simulink model "HMI_C_S_28379D_071224_FW"  (R2024b)
settings: Solver=ode4  StartTime=0.0  StopTime=Inf  FixedStep=Ts  RelTol=1e-3  EnableMultiTasking=on
InitFcn:
  | Ts=1e-4
model workspace (MAT data in the model file):
  encoderResolution = 2000
  hallOffset = '0.5'
  indexOffset = 850
  polePairs = '4'
libraries: simulink x4, c2837xDlib x2, c280xlib x2
settings Model: ExtModeTrigDuration=8  Creator=matti  LastModifiedBy=Administrator
settings SolverCC: AlgebraicLoopSolver=TrustRegion
settings DataIOCC: LimitDataPoints=on  SaveFormat=Array  SignalLoggingSaveFormat=ModelDataLogs  SaveOutput=off  SaveTime=off  ReturnWorkspaceOutputs=off
settings OptimizationCC: DefaultUnderspecifiedDataType=single  OptimizeBlockIOStorage=off  BufferReuse=off  GlobalBufferReuse=off  ExpressionFolding=off  ExpressionDepthLimit=2147483647  LocalBlockOutputs=off  InitFltsAndDblsToZero=on  NoFixptDivByZeroProtection=on  EfficientFloat2IntCast=on  EfficientMapNaN2IntZero=off  LifeSpan=Inf  MaxStackSize=1024  OptimizeDataStoreBuffers=off  BusAssignmentInplaceUpdate=off  EfficientTunableParamExpr=on
settings DebuggingCC: ReadBeforeWriteMsg=DisableAll  WriteAfterWriteMsg=DisableAll  WriteAfterReadMsg=DisableAll  CheckSSInitialOutputMsg=off  UnderspecifiedInitializationDetection=Classic  MergeDetectMultiDrivingBlocksExec=none  SignalResolutionControl=TryResolveAllWithWarning  SolverPrmCheckMsg=warning  InheritedTsInSrcMsg=none  MultiTaskDSMMsg=none  MultiTaskCondExecSysMsg=none  TasksWithSamePriorityMsg=none  SigSpecEnsureSampleTimeMsg=none  IntegerOverflowMsg=none  ParameterPrecisionLossMsg=none  FcnCallInpInsideContextMsg=warning  UnconnectedInputMsg=warning  UnconnectedOutputMsg=warning  UnconnectedLineMsg=warning  StateNameClashWarn=warning  SFUnexpectedBacktrackingDiag=warning  SFNoUnconditionalDefaultTransitionDiag=warning  SFExecutionAtInitializationDiag=none  IntegerSaturationMsg=none  ArithmeticOperatorsInVariantConditions=warning
settings HardwareCC: ProdBitPerChar=16  ProdBitPerInt=16  ProdBitPerPointer=32  ProdBitPerSizeT=32  ProdBitPerPtrDiffT=32  ProdLargestAtomicInteger=Integer  ProdLargestAtomicFloat=None  ProdWordSize=16  ProdLongLongMode=on  ProdHWDeviceType=Texas Instruments->C2000  TargetBitPerChar=16  TargetBitPerInt=16  TargetBitPerPointer=16  TargetLargestAtomicInteger=Integer  TargetIntDivRoundTo=Zero  TargetEndianess=LittleEndian  TargetWordSize=16  TargetHWDeviceType=TI C2000  HardwareBoardFeatureSet=SoCBlockset
settings ModelReferenceCC: EnableRefExpFcnMdlSchedulingChecks=on  PropagateSignalLabelsOutOfModel=off
settings SFSimCC: SimUseLocalCustomCode=off  MATLABDynamicMemAlloc=off  CustomCodeUndefinedFunction=UseInterfaceOnly
settings RTWCC: Description=Embedded Coder  SystemTargetFile=ert.tlc  HardwareBoard=TI Delfino F28379D LaunchPad  TemplateMakefile=ert_default_tmf  GenerateReport=on  RTWUseLocalCustomCode=off  CustomHeaderCode=#include<stdlib.h>  Toolchain=Texas Instruments Code Composer Studio (C2000)  IncludeHyperlinkInReport=on  LaunchReport=on  CodeProfilingSaveOptions=MetricsOnly  GenerateTraceInfo=on  GenerateTraceReport=on  GenerateTraceReportSl=on  GenerateTraceReportSf=on  GenerateTraceReportEml=on  GPUComputeCapability=3.5
settings CodeAppCC: IgnoreCustomStorageClasses=off  CustomSymbolStrType=$N$R$M  StateflowObjectComments=on  InternalIdentifier=Classic
settings ERTTargetCC: CodeReplacementLibrary=TI C28x  MultiwordLength=2048  SupportContinuousTime=on  ExtModeTransport=4  ExtModeStaticAlloc=on  ExtModeAutomaticAllocSize=off  ExtModeStaticAllocSize=10000  ExtModeMexFile=ext_xcp  ExtModeIntrfLevel=Level2 - Open  InlinedParameterPlacement=Hierarchical  ConvertIfToSwitch=off  SuppressUnreachableDefaultCases=off  MemSecPackage=tic2000demospkg  MemSecFuncExecute=code_ramfuncs  DynamicArrayContainerType=coder::array
settings ConfigComp: CovMetricSettings=dw  CovSaveCumulativeToWorkspaceVar=on  CovSaveSingleToWorkspaceVar=on  CovExternalEMLEnable=off  CovSFcnEnable=off
settings SimscapeCC: SimscapeNormalizeSystem=off

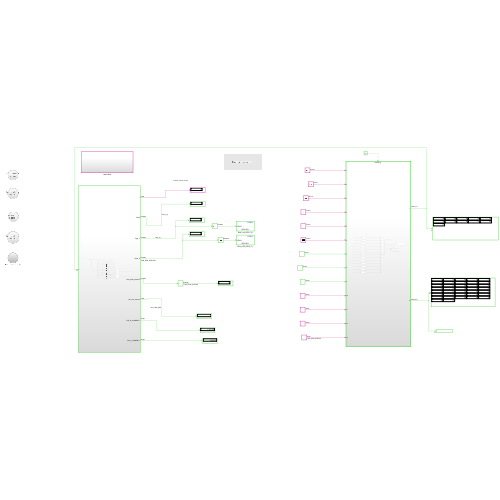
[thumbnail: Simulink's stored preview of the top-level diagram]
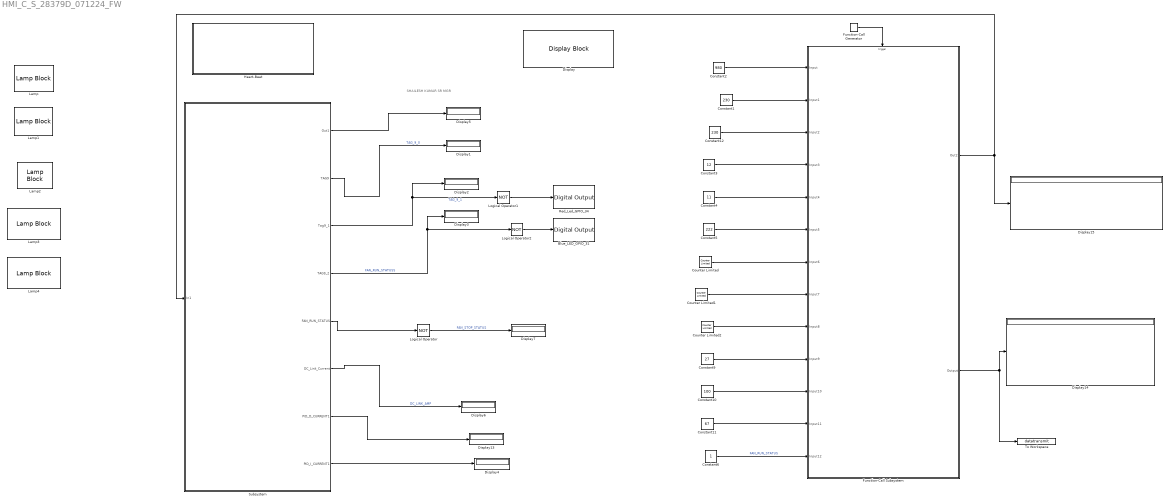
== system HMI_C_S_28379D_071224_FW ==
  note: SHAILESH KUMAR SR MGR
  Blue_LED_GPIO_31 : c2837xDlib/Digital Output  GPIO_Number=GPIO24~GPIO31  GPIO_Bit0=off  GPIO_BIT0_Toggle=off  GPIO_Bit1=off  GPIO_BIT1_Toggle=off  GPIO_Bit2=off  GPIO_BIT2_Toggle=off  GPIO_Bit3=off  GPIO_BIT3_Toggle=off  GPIO_Bit4=off  GPIO_BIT4_Toggle=off  GPIO_Bit5=off  GPIO_BIT5_Toggle=off  GPIO_Bit6=off  GPIO_BIT6_Toggle=off  GPIO_Bit7=on  GPIO_BIT7_Toggle=off
  Constant1 : Constant  Value=230  OutDataTypeStr=uint16
  Constant10 : Constant  Value=100  OutDataTypeStr=uint16
  Constant11 : Constant  Value=67  OutDataTypeStr=uint16
  Constant12 : Constant  Value=230  OutDataTypeStr=uint16
  Constant2 : Constant  Value=980  OutDataTypeStr=uint16
  Constant3 : Constant  Value=12  OutDataTypeStr=uint16
  Constant4 : Constant  Value=11  OutDataTypeStr=uint16
  Constant5 : Constant  Value=222  OutDataTypeStr=uint16
  Constant6 : Constant  OutDataTypeStr=uint8
  Constant9 : Constant  Value=27  OutDataTypeStr=uint16
  Counter Limited : simulink/Sources/Counter Limited  uplimit=999  tsamp=-1
  Counter Limited1 : simulink/Sources/Counter Limited  uplimit=999  tsamp=-1
  Counter Limited2 : simulink/Sources/Counter Limited  uplimit=999  tsamp=-1
  Display : DisplayBlock  Transparency=1
  Display{1..7,13..15} (10 alike) : Display
  Function-Call Generator : simulink/Ports & Subsystems/Function-Call Generator  sample_time=0.1  numberOfIterations=1  DisallowWideOutput=off
  Function-Call Subsystem : Subsystem  TreatAsAtomicUnit=on
  Heart-Beat : Subsystem
  Lamp : LampBlock
  Lamp1 : LampBlock
  Lamp2 : LampBlock
  Lamp3 : LampBlock  LabelPosition=Bottom
  Lamp4 : LampBlock  LabelPosition=Bottom
  Logical Operator : Logic  Operator=NOT  AllPortsSameDT=off  OutDataTypeStr=boolean
  Logical Operator1 : Logic  Operator=NOT  AllPortsSameDT=off  OutDataTypeStr=boolean
  Logical Operator2 : Logic  Operator=NOT  AllPortsSameDT=off  OutDataTypeStr=boolean
  Red_Led_GPIO_34 : c2837xDlib/Digital Output  GPIO_Number=GPIO32~GPIO39  GPIO_Bit0=off  GPIO_BIT0_Toggle=off  GPIO_Bit1=off  GPIO_BIT1_Toggle=off  GPIO_Bit2=on  GPIO_BIT2_Toggle=off  GPIO_Bit3=off  GPIO_BIT3_Toggle=off  GPIO_Bit4=off  GPIO_BIT4_Toggle=off  GPIO_Bit5=off  GPIO_BIT5_Toggle=off  GPIO_Bit6=off  GPIO_BIT6_Toggle=off  GPIO_Bit7=off  GPIO_BIT7_Toggle=off
  Subsystem : Subsystem
  To Workspace : ToWorkspace  VariableName=datatransmit  SampleTime=-1
      settings: Save2DSignal=2-D array (concatenate along first dimension)
  wires:
  Subsystem/1(Out1) -> Display5/1
  Subsystem/3(Tag9_1) -> Display2/1, Logical Operator1/1  "TAG_9_1"
  Subsystem/6(DC_Link_Current) -> Display6/1  "DC_LINK_AMP"
  Subsystem/2(TAG9) -> Display1/1  "TAG_9_0"
  Logical Operator/1 -> Display7/1  "FAN_STOP_STATUS"
  Function-Call Generator/1 -> Function-Call Subsystem/Trigger
  Function-Call Subsystem/1(Out2) -> Subsystem/1(In1), Display15/1
  Constant2/1 -> Function-Call Subsystem/1(Input)
  Constant1/1 -> Function-Call Subsystem/2(Input1)
  Constant12/1 -> Function-Call Subsystem/3(Input2)
  Constant3/1 -> Function-Call Subsystem/4(Input3)
  Constant4/1 -> Function-Call Subsystem/5(Input4)
  Constant5/1 -> Function-Call Subsystem/6(Input5)
  Counter Limited/1 -> Function-Call Subsystem/7(Input6)
  Counter Limited1/1 -> Function-Call Subsystem/8(Input7)
  Counter Limited2/1 -> Function-Call Subsystem/9(Input8)
  Constant9/1 -> Function-Call Subsystem/10(Input9)
  Constant10/1 -> Function-Call Subsystem/11(Input10)
  Constant11/1 -> Function-Call Subsystem/12(Input11)
  Constant6/1 -> Function-Call Subsystem/13(Input12)  "FAN_RUN_STATUS"
  Function-Call Subsystem/2(Output) -> To Workspace/1, Display14/1
  Logical Operator1/1 -> Red_Led_GPIO_34/1
  Logical Operator2/1 -> Blue_LED_GPIO_31/1
  Subsystem/4(TAG9_2) -> Display3/1, Logical Operator2/1  "FAN_RUN_STATUSS"
  Subsystem/5(FAN_RUN_STATUS) -> Logical Operator/1
  Subsystem/7(PID_D_CURRENT1) -> Display13/1
  Subsystem/8(PID_I_CURRENT1) -> Display4/1

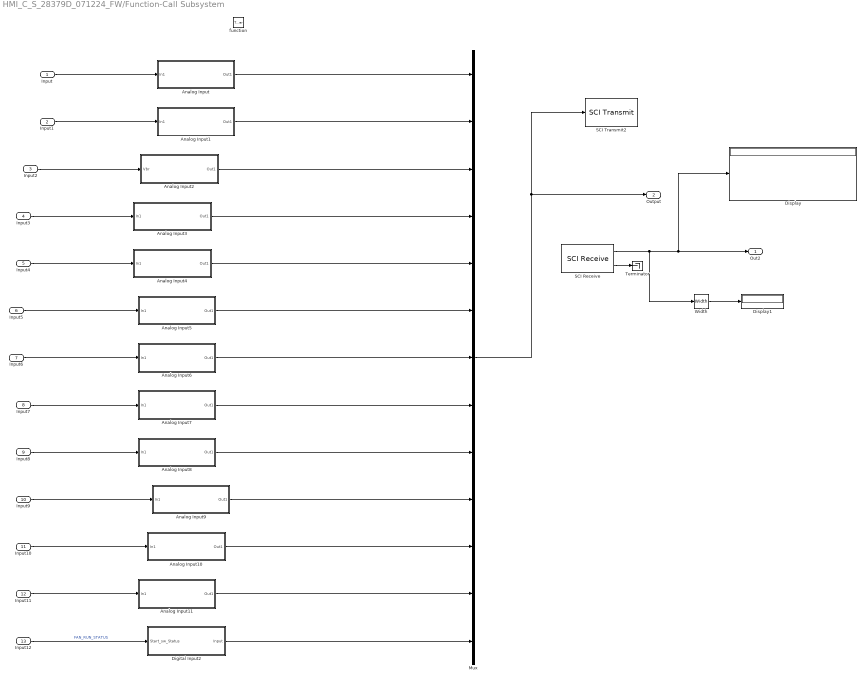
== system HMI_C_S_28379D_071224_FW/Function-Call Subsystem ==
  Input : Inport
  Input1 : Inport  Port=2
  Input2 : Inport  Port=3
  Input3 : Inport  Port=4
  Input4 : Inport  Port=5
  Input5 : Inport  Port=6
  Input6 : Inport  Port=7
  Input7 : Inport  Port=8
  Input8 : Inport  Port=9
  Input9 : Inport  Port=10
  Input10 : Inport  Port=11
  Input11 : Inport  Port=12
  Input12 : Inport  Port=13
  function : TriggerPort  TriggerType=function-call  VariantControl=(inherit)
  Analog Input : Subsystem
  Analog Input1 : Subsystem
  Analog Input10 : Subsystem
  Analog Input11 : Subsystem
  Analog Input2 : Subsystem
  Analog Input3 : Subsystem
  Analog Input4 : Subsystem
  Analog Input5 : Subsystem
  Analog Input6 : Subsystem
  Analog Input7 : Subsystem
  Analog Input8 : Subsystem
  Analog Input9 : Subsystem
  Digital Input2 : Subsystem
  Display : Display
  Display1 : Display
  Mux : Mux  Inputs=13
  SCI Receive : c280xlib/SCI Receive  Priority=2  sciModule=B  dataHead='S'  headerCheckMaxCount=16  dataTail='E'  dataType=uint8  dataLenOptions=Length via dialog  dataDim=11  maxDataLength=1  initValue=0  errOption=Output the last received value  errValue=0  sampleTime=-1  blockingMode=off  timeOut=inf  outputStatus=on
      settings: LibrarySourceBlock=c2837xDlib/SCI Receive
  SCI Transmit2 : c280xlib/SCI Transmit  sciModule=B  dataHead='S'  dataTail='E'  frameSize=[1 37]  blockingMode=on  outputStatus=off
      settings: LibrarySourceBlock=c2837xDlib/SCI Transmit
  Terminator : Terminator
  Width : Width  DataType=uint8
  Out2 : Outport
  Output : Outport  Port=2
  wires:
  SCI Receive/1 -> Width/1, Display/1, Out2/1
  SCI Receive/2 -> Terminator/1
  Analog Input1/1(Out1) -> Mux/2
  Analog Input2/1(Out1) -> Mux/3
  Analog Input9/1(Out1) -> Mux/10
  Analog Input7/1(Out1) -> Mux/8
  Analog Input4/1(Out1) -> Mux/5
  Analog Input5/1(Out1) -> Mux/6
  Digital Input2/1(Input) -> Mux/13
  Analog Input8/1(Out1) -> Mux/9
  Analog Input10/1(Out1) -> Mux/11
  Analog Input11/1(Out1) -> Mux/12
  Analog Input/1(Out1) -> Mux/1
  Input1/1 -> Analog Input1/1(In1)
  Input2/1 -> Analog Input2/1(Vbr)
  Input/1 -> Analog Input/1(In1)
  Input9/1 -> Analog Input9/1(In1)
  Input12/1 -> Digital Input2/1(Start_sw_Status)  "FAN_RUN_STATUS"
  Analog Input3/1(Out1) -> Mux/4
  Input11/1 -> Analog Input11/1(In1)
  Analog Input6/1(Out1) -> Mux/7
  Input10/1 -> Analog Input10/1(In1)
  Mux/1 -> SCI Transmit2/1, Output/1
  Input3/1 -> Analog Input3/1(In1)
  Input4/1 -> Analog Input4/1(In1)
  Input5/1 -> Analog Input5/1(In1)
  Input6/1 -> Analog Input6/1(In1)
  Input7/1 -> Analog Input7/1(In1)
  Input8/1 -> Analog Input8/1(In1)
  Width/1 -> Display1/1

== system HMI_C_S_28379D_071224_FW/Heart-Beat ==

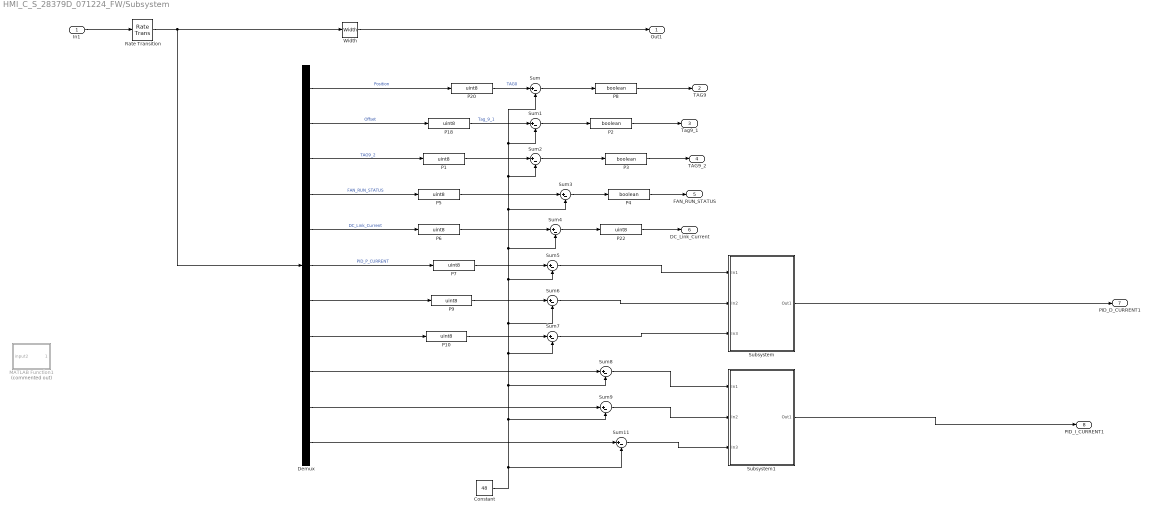
== system HMI_C_S_28379D_071224_FW/Subsystem ==
  In1 : Inport
  Constant : Constant  Value=48  OutDataTypeStr=uint8
  Demux : Demux  Outputs=11
  MATLAB Function1 : MATLAB Function  Commented=on  TreatAsAtomicUnit=on
  P{1,5..7,9..10,18,20,22} (9 alike) : DataTypeConversion  OutDataTypeStr=uint8  SaturateOnIntegerOverflow=off  RndMeth=Floor
  P{2..4,8} (4 alike) : DataTypeConversion  OutDataTypeStr=boolean  SaturateOnIntegerOverflow=off  RndMeth=Floor
  Rate Transition : RateTransition
  Subsystem : Subsystem
  Subsystem1 : Subsystem
  Sum{,1..9,11} (11 alike) : Sum  Inputs=|+-
  Width : Width  DataType=uint8
  Out1 : Outport
  TAG9 : Outport  Port=2
  Tag9_1 : Outport  Port=3
  TAG9_2 : Outport  Port=4
  FAN_RUN_STATUS : Outport  Port=5
  DC_Link_Current : Outport  Port=6
  PID_D_CURRENT1 : Outport  Port=7
  PID_I_CURRENT1 : Outport  Port=8
  wires:
  Demux/1 -> P20/1  "Position"
  P1/1 -> Sum2/1
  P3/1 -> TAG9_2/1
  Sum1/1 -> P2/1
  P10/1 -> Sum7/1
  P2/1 -> Tag9_1/1
  Sum/1 -> P8/1
  P18/1 -> Sum1/1  "Tag_9_1"
  P6/1 -> Sum4/1
  P9/1 -> Sum6/1
  P7/1 -> Sum5/1
  Demux/5 -> P6/1  "DC_Link_Current"
  Demux/6 -> P7/1  "PID_P_CURRENT"
  Demux/8 -> P10/1
  P4/1 -> FAN_RUN_STATUS/1
  Demux/4 -> P5/1  "FAN_RUN_STATUS"
  P5/1 -> Sum3/1
  Sum3/1 -> P4/1
  Demux/3 -> P1/1  "TAG9_2"
  Sum4/1 -> P22/1
  Demux/2 -> P18/1  "Offset"
  Sum2/1 -> P3/1
  In1/1 -> Rate Transition/1
  Width/1 -> Out1/1
  P20/1 -> Sum/1  "TAG0"
  Rate Transition/1 -> Demux/1, Width/1
  Demux/7 -> P9/1
  P8/1 -> TAG9/1
  P22/1 -> DC_Link_Current/1
  Constant/1 -> Sum11/2, Sum9/2, Sum8/2, Sum7/2, Sum6/2, Sum5/2, Sum4/2, Sum3/2, Sum2/2, Sum1/2, Sum/2
  Sum5/1 -> Subsystem/1(In1)
  Sum6/1 -> Subsystem/2(In2)
  Sum7/1 -> Subsystem/3(In3)
  Subsystem/1(Out1) -> PID_D_CURRENT1/1
  Demux/9 -> Sum8/1
  Demux/10 -> Sum9/1
  Demux/11 -> Sum11/1
  Sum11/1 -> Subsystem1/3(In3)
  Sum9/1 -> Subsystem1/2(In2)
  Sum8/1 -> Subsystem1/1(In1)
  Subsystem1/1(Out1) -> PID_I_CURRENT1/1

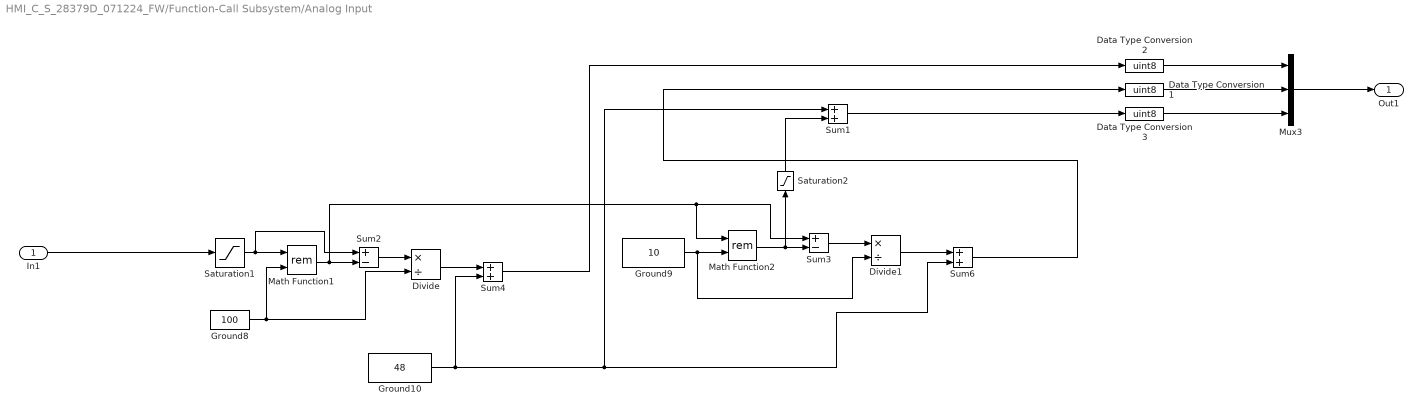
== system HMI_C_S_28379D_071224_FW/Function-Call Subsystem/Analog Input ==
  In1 : Inport
  Data Type Conversion1 : DataTypeConversion  OutDataTypeStr=uint8  SaturateOnIntegerOverflow=off  RndMeth=Floor
  Data Type Conversion2 : DataTypeConversion  OutDataTypeStr=uint8  SaturateOnIntegerOverflow=off  RndMeth=Floor
  Data Type Conversion3 : DataTypeConversion  OutDataTypeStr=uint8  SaturateOnIntegerOverflow=off  RndMeth=Floor
  Divide : Product  Inputs=*/  OutDataTypeStr=int16
  Divide1 : Product  Inputs=*/  OutDataTypeStr=int16
  Ground10 : Constant  Value=48  OutDataTypeStr=int16
  Ground8 : Constant  Value=100  OutDataTypeStr=int16
  Ground9 : Constant  Value=10  OutDataTypeStr=int16
  Math Function1 : Math  Operator=rem  SignedPower=on
  Math Function2 : Math  Operator=rem  SignedPower=on
  Mux3 : Mux  Inputs=3
  Saturation1 : Saturate  UpperLimit=999  LowerLimit=0  OutDataTypeStr=int16
  Saturation2 : Saturate  UpperLimit=9  LowerLimit=0
  Sum1 : Sum  OutDataTypeStr=uint8
  Sum2 : Sum  Inputs=+-  OutDataTypeStr=double
  Sum3 : Sum  Inputs=+-
  Sum4 : Sum  OutDataTypeStr=uint8
  Sum6 : Sum  OutDataTypeStr=uint8
  Out1 : Outport
  wires:
  Saturation1/1 -> Sum2/1, Math Function1/1
  Ground8/1 -> Divide/2, Math Function1/2
  Sum4/1 -> Data Type Conversion2/1
  Sum1/1 -> Data Type Conversion3/1
  Divide/1 -> Sum4/1
  Divide1/1 -> Sum6/1
  Sum2/1 -> Divide/1
  In1/1 -> Saturation1/1
  Data Type Conversion2/1 -> Mux3/1
  Mux3/1 -> Out1/1
  Data Type Conversion3/1 -> Mux3/3
  Data Type Conversion1/1 -> Mux3/2
  Math Function1/1 -> Sum2/2, Math Function2/1, Sum3/1
  Sum3/1 -> Divide1/1
  Sum6/1 -> Data Type Conversion1/1
  Ground10/1 -> Sum4/2, Sum6/2, Sum1/1
  Ground9/1 -> Divide1/2, Math Function2/2
  Math Function2/1 -> Sum3/2, Saturation2/1
  Saturation2/1 -> Sum1/2

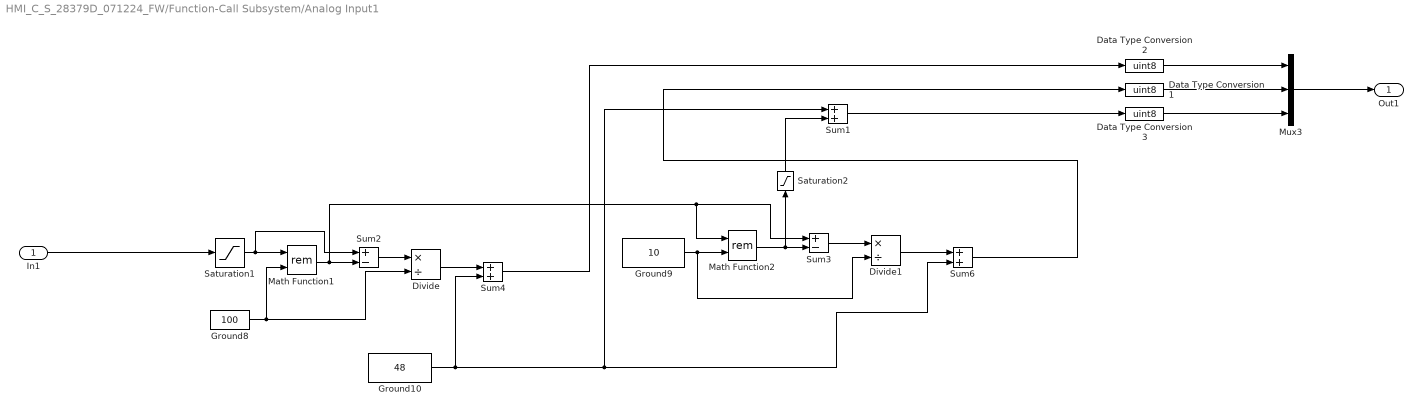
== system HMI_C_S_28379D_071224_FW/Function-Call Subsystem/Analog Input1 ==
  In1 : Inport
  Data Type Conversion1 : DataTypeConversion  OutDataTypeStr=uint8  SaturateOnIntegerOverflow=off  RndMeth=Floor
  Data Type Conversion2 : DataTypeConversion  OutDataTypeStr=uint8  SaturateOnIntegerOverflow=off  RndMeth=Floor
  Data Type Conversion3 : DataTypeConversion  OutDataTypeStr=uint8  SaturateOnIntegerOverflow=off  RndMeth=Floor
  Divide : Product  Inputs=*/  OutDataTypeStr=int16
  Divide1 : Product  Inputs=*/  OutDataTypeStr=int16
  Ground10 : Constant  Value=48  OutDataTypeStr=int16
  Ground8 : Constant  Value=100  OutDataTypeStr=int16
  Ground9 : Constant  Value=10  OutDataTypeStr=int16
  Math Function1 : Math  Operator=rem  SignedPower=on
  Math Function2 : Math  Operator=rem  SignedPower=on
  Mux3 : Mux  Inputs=3
  Saturation1 : Saturate  UpperLimit=999  LowerLimit=0  OutDataTypeStr=int16
  Saturation2 : Saturate  UpperLimit=9  LowerLimit=0
  Sum1 : Sum  OutDataTypeStr=uint8
  Sum2 : Sum  Inputs=+-  OutDataTypeStr=double
  Sum3 : Sum  Inputs=+-
  Sum4 : Sum  OutDataTypeStr=uint8
  Sum6 : Sum  OutDataTypeStr=uint8
  Out1 : Outport
  wires:
  Saturation1/1 -> Sum2/1, Math Function1/1
  Ground8/1 -> Divide/2, Math Function1/2
  Sum4/1 -> Data Type Conversion2/1
  Sum1/1 -> Data Type Conversion3/1
  Divide/1 -> Sum4/1
  Divide1/1 -> Sum6/1
  Sum2/1 -> Divide/1
  In1/1 -> Saturation1/1
  Data Type Conversion2/1 -> Mux3/1
  Mux3/1 -> Out1/1
  Data Type Conversion3/1 -> Mux3/3
  Data Type Conversion1/1 -> Mux3/2
  Math Function1/1 -> Sum2/2, Math Function2/1, Sum3/1
  Sum3/1 -> Divide1/1
  Sum6/1 -> Data Type Conversion1/1
  Ground10/1 -> Sum4/2, Sum6/2, Sum1/1
  Ground9/1 -> Divide1/2, Math Function2/2
  Math Function2/1 -> Sum3/2, Saturation2/1
  Saturation2/1 -> Sum1/2

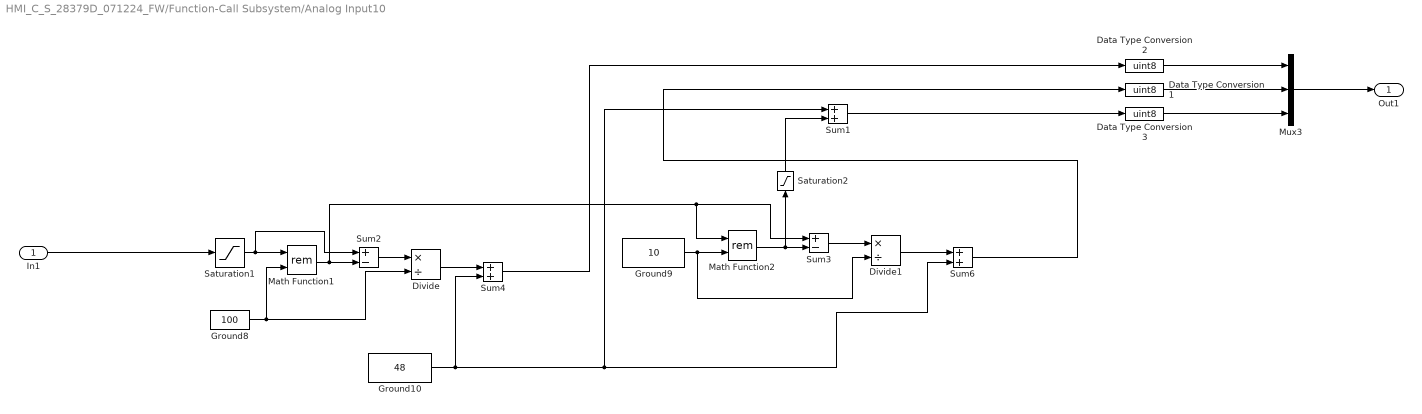
== system HMI_C_S_28379D_071224_FW/Function-Call Subsystem/Analog Input10 ==
  In1 : Inport
  Data Type Conversion1 : DataTypeConversion  OutDataTypeStr=uint8  SaturateOnIntegerOverflow=off  RndMeth=Floor
  Data Type Conversion2 : DataTypeConversion  OutDataTypeStr=uint8  SaturateOnIntegerOverflow=off  RndMeth=Floor
  Data Type Conversion3 : DataTypeConversion  OutDataTypeStr=uint8  SaturateOnIntegerOverflow=off  RndMeth=Floor
  Divide : Product  Inputs=*/  OutDataTypeStr=int16
  Divide1 : Product  Inputs=*/  OutDataTypeStr=int16
  Ground10 : Constant  Value=48  OutDataTypeStr=int16
  Ground8 : Constant  Value=100  OutDataTypeStr=int16
  Ground9 : Constant  Value=10  OutDataTypeStr=int16
  Math Function1 : Math  Operator=rem  SignedPower=on
  Math Function2 : Math  Operator=rem  SignedPower=on
  Mux3 : Mux  Inputs=3
  Saturation1 : Saturate  UpperLimit=999  LowerLimit=0  OutDataTypeStr=int16
  Saturation2 : Saturate  UpperLimit=9  LowerLimit=0
  Sum1 : Sum  OutDataTypeStr=uint8
  Sum2 : Sum  Inputs=+-  OutDataTypeStr=double
  Sum3 : Sum  Inputs=+-
  Sum4 : Sum  OutDataTypeStr=uint8
  Sum6 : Sum  OutDataTypeStr=uint8
  Out1 : Outport
  wires:
  Saturation1/1 -> Sum2/1, Math Function1/1
  Ground8/1 -> Divide/2, Math Function1/2
  Sum4/1 -> Data Type Conversion2/1
  Sum1/1 -> Data Type Conversion3/1
  Divide/1 -> Sum4/1
  Divide1/1 -> Sum6/1
  Sum2/1 -> Divide/1
  In1/1 -> Saturation1/1
  Data Type Conversion2/1 -> Mux3/1
  Mux3/1 -> Out1/1
  Data Type Conversion3/1 -> Mux3/3
  Data Type Conversion1/1 -> Mux3/2
  Math Function1/1 -> Sum2/2, Math Function2/1, Sum3/1
  Sum3/1 -> Divide1/1
  Sum6/1 -> Data Type Conversion1/1
  Ground10/1 -> Sum4/2, Sum6/2, Sum1/1
  Ground9/1 -> Divide1/2, Math Function2/2
  Math Function2/1 -> Sum3/2, Saturation2/1
  Saturation2/1 -> Sum1/2

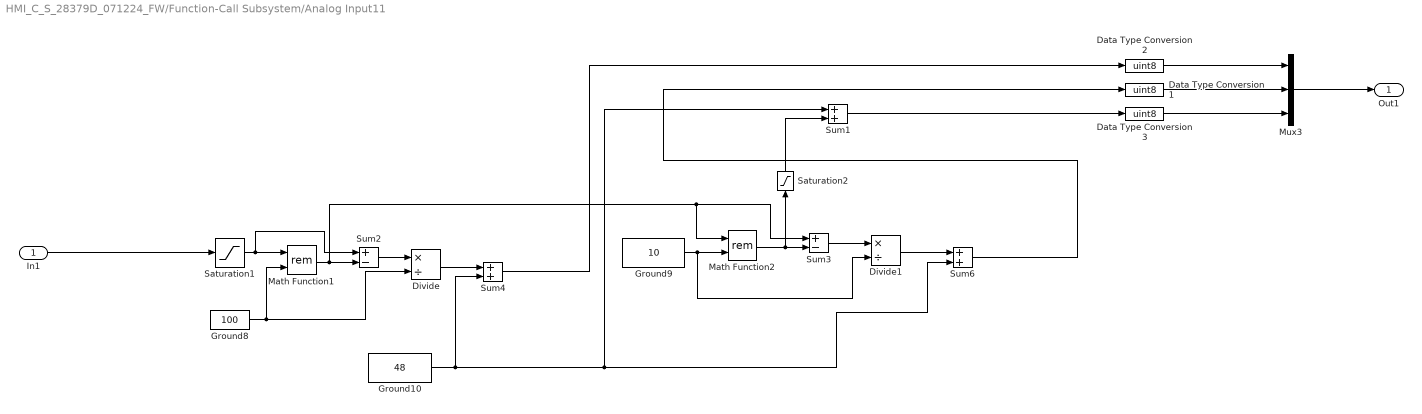
== system HMI_C_S_28379D_071224_FW/Function-Call Subsystem/Analog Input11 ==
  In1 : Inport
  Data Type Conversion1 : DataTypeConversion  OutDataTypeStr=uint8  SaturateOnIntegerOverflow=off  RndMeth=Floor
  Data Type Conversion2 : DataTypeConversion  OutDataTypeStr=uint8  SaturateOnIntegerOverflow=off  RndMeth=Floor
  Data Type Conversion3 : DataTypeConversion  OutDataTypeStr=uint8  SaturateOnIntegerOverflow=off  RndMeth=Floor
  Divide : Product  Inputs=*/  OutDataTypeStr=int16
  Divide1 : Product  Inputs=*/  OutDataTypeStr=int16
  Ground10 : Constant  Value=48  OutDataTypeStr=int16
  Ground8 : Constant  Value=100  OutDataTypeStr=int16
  Ground9 : Constant  Value=10  OutDataTypeStr=int16
  Math Function1 : Math  Operator=rem  SignedPower=on
  Math Function2 : Math  Operator=rem  SignedPower=on
  Mux3 : Mux  Inputs=3
  Saturation1 : Saturate  UpperLimit=999  LowerLimit=0  OutDataTypeStr=int16
  Saturation2 : Saturate  UpperLimit=9  LowerLimit=0
  Sum1 : Sum  OutDataTypeStr=uint8
  Sum2 : Sum  Inputs=+-  OutDataTypeStr=double
  Sum3 : Sum  Inputs=+-
  Sum4 : Sum  OutDataTypeStr=uint8
  Sum6 : Sum  OutDataTypeStr=uint8
  Out1 : Outport
  wires:
  Saturation1/1 -> Sum2/1, Math Function1/1
  Ground8/1 -> Divide/2, Math Function1/2
  Sum4/1 -> Data Type Conversion2/1
  Sum1/1 -> Data Type Conversion3/1
  Divide/1 -> Sum4/1
  Divide1/1 -> Sum6/1
  Sum2/1 -> Divide/1
  In1/1 -> Saturation1/1
  Data Type Conversion2/1 -> Mux3/1
  Mux3/1 -> Out1/1
  Data Type Conversion3/1 -> Mux3/3
  Data Type Conversion1/1 -> Mux3/2
  Math Function1/1 -> Sum2/2, Math Function2/1, Sum3/1
  Sum3/1 -> Divide1/1
  Sum6/1 -> Data Type Conversion1/1
  Ground10/1 -> Sum4/2, Sum6/2, Sum1/1
  Ground9/1 -> Divide1/2, Math Function2/2
  Math Function2/1 -> Sum3/2, Saturation2/1
  Saturation2/1 -> Sum1/2

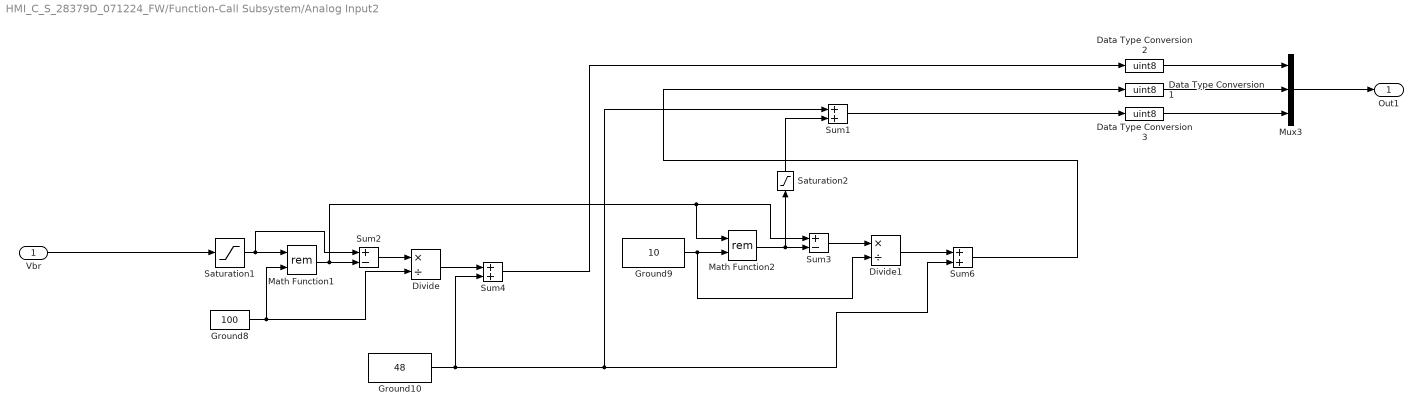
== system HMI_C_S_28379D_071224_FW/Function-Call Subsystem/Analog Input2 ==
  Vbr : Inport
  Data Type Conversion1 : DataTypeConversion  OutDataTypeStr=uint8  SaturateOnIntegerOverflow=off  RndMeth=Floor
  Data Type Conversion2 : DataTypeConversion  OutDataTypeStr=uint8  SaturateOnIntegerOverflow=off  RndMeth=Floor
  Data Type Conversion3 : DataTypeConversion  OutDataTypeStr=uint8  SaturateOnIntegerOverflow=off  RndMeth=Floor
  Divide : Product  Inputs=*/  OutDataTypeStr=int16
  Divide1 : Product  Inputs=*/  OutDataTypeStr=int16
  Ground10 : Constant  Value=48  OutDataTypeStr=int16
  Ground8 : Constant  Value=100  OutDataTypeStr=int16
  Ground9 : Constant  Value=10  OutDataTypeStr=int16
  Math Function1 : Math  Operator=rem  SignedPower=on
  Math Function2 : Math  Operator=rem  SignedPower=on
  Mux3 : Mux  Inputs=3
  Saturation1 : Saturate  UpperLimit=999  LowerLimit=0  OutDataTypeStr=int16
  Saturation2 : Saturate  UpperLimit=9  LowerLimit=0
  Sum1 : Sum  OutDataTypeStr=uint8
  Sum2 : Sum  Inputs=+-  OutDataTypeStr=double
  Sum3 : Sum  Inputs=+-
  Sum4 : Sum  OutDataTypeStr=uint8
  Sum6 : Sum  OutDataTypeStr=uint8
  Out1 : Outport
  wires:
  Saturation1/1 -> Sum2/1, Math Function1/1
  Ground8/1 -> Divide/2, Math Function1/2
  Sum4/1 -> Data Type Conversion2/1
  Sum1/1 -> Data Type Conversion3/1
  Divide/1 -> Sum4/1
  Divide1/1 -> Sum6/1
  Sum2/1 -> Divide/1
  Vbr/1 -> Saturation1/1
  Data Type Conversion2/1 -> Mux3/1
  Mux3/1 -> Out1/1
  Data Type Conversion3/1 -> Mux3/3
  Data Type Conversion1/1 -> Mux3/2
  Math Function1/1 -> Sum2/2, Math Function2/1, Sum3/1
  Sum3/1 -> Divide1/1
  Sum6/1 -> Data Type Conversion1/1
  Ground10/1 -> Sum4/2, Sum6/2, Sum1/1
  Ground9/1 -> Divide1/2, Math Function2/2
  Math Function2/1 -> Sum3/2, Saturation2/1
  Saturation2/1 -> Sum1/2

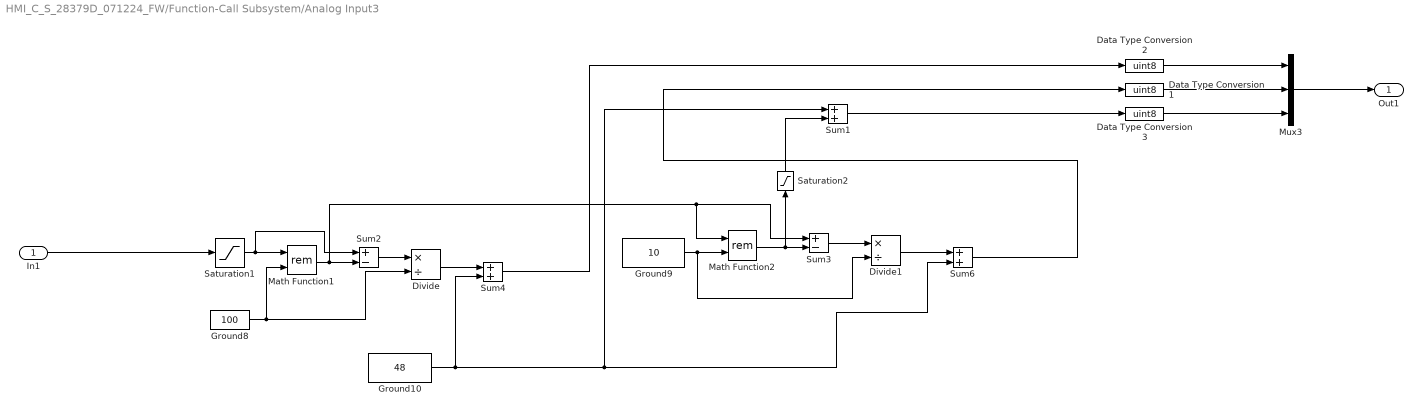
== system HMI_C_S_28379D_071224_FW/Function-Call Subsystem/Analog Input3 ==
  In1 : Inport
  Data Type Conversion1 : DataTypeConversion  OutDataTypeStr=uint8  SaturateOnIntegerOverflow=off  RndMeth=Floor
  Data Type Conversion2 : DataTypeConversion  OutDataTypeStr=uint8  SaturateOnIntegerOverflow=off  RndMeth=Floor
  Data Type Conversion3 : DataTypeConversion  OutDataTypeStr=uint8  SaturateOnIntegerOverflow=off  RndMeth=Floor
  Divide : Product  Inputs=*/  OutDataTypeStr=int16
  Divide1 : Product  Inputs=*/  OutDataTypeStr=int16
  Ground10 : Constant  Value=48  OutDataTypeStr=int16
  Ground8 : Constant  Value=100  OutDataTypeStr=int16
  Ground9 : Constant  Value=10  OutDataTypeStr=int16
  Math Function1 : Math  Operator=rem  SignedPower=on
  Math Function2 : Math  Operator=rem  SignedPower=on
  Mux3 : Mux  Inputs=3
  Saturation1 : Saturate  UpperLimit=999  LowerLimit=0  OutDataTypeStr=int16
  Saturation2 : Saturate  UpperLimit=9  LowerLimit=0
  Sum1 : Sum  OutDataTypeStr=uint8
  Sum2 : Sum  Inputs=+-  OutDataTypeStr=double
  Sum3 : Sum  Inputs=+-
  Sum4 : Sum  OutDataTypeStr=uint8
  Sum6 : Sum  OutDataTypeStr=uint8
  Out1 : Outport
  wires:
  Saturation1/1 -> Sum2/1, Math Function1/1
  Ground8/1 -> Divide/2, Math Function1/2
  Sum4/1 -> Data Type Conversion2/1
  Sum1/1 -> Data Type Conversion3/1
  Divide/1 -> Sum4/1
  Divide1/1 -> Sum6/1
  Sum2/1 -> Divide/1
  In1/1 -> Saturation1/1
  Data Type Conversion2/1 -> Mux3/1
  Mux3/1 -> Out1/1
  Data Type Conversion3/1 -> Mux3/3
  Data Type Conversion1/1 -> Mux3/2
  Math Function1/1 -> Sum2/2, Math Function2/1, Sum3/1
  Sum3/1 -> Divide1/1
  Sum6/1 -> Data Type Conversion1/1
  Ground10/1 -> Sum4/2, Sum6/2, Sum1/1
  Ground9/1 -> Divide1/2, Math Function2/2
  Math Function2/1 -> Sum3/2, Saturation2/1
  Saturation2/1 -> Sum1/2

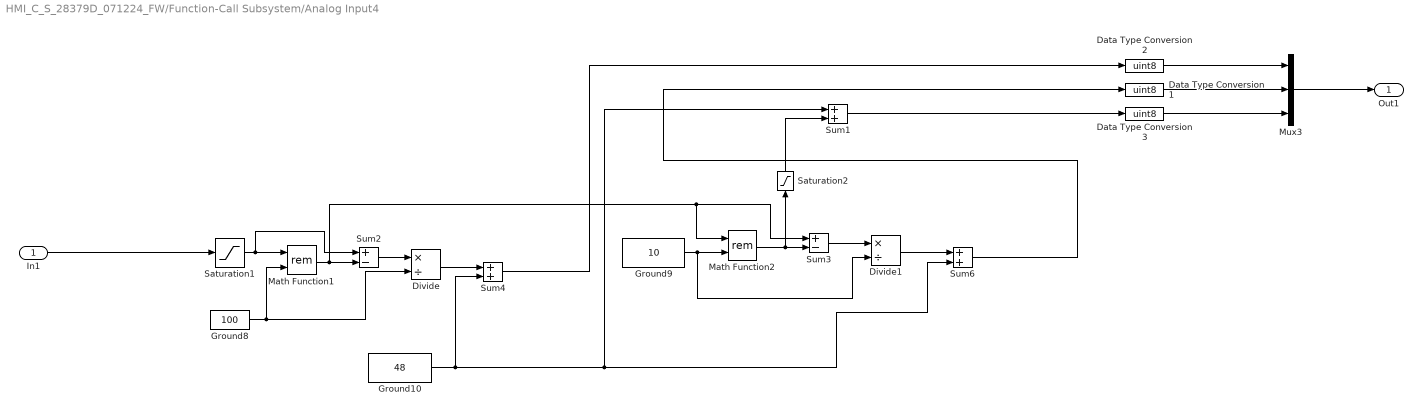
== system HMI_C_S_28379D_071224_FW/Function-Call Subsystem/Analog Input4 ==
  In1 : Inport
  Data Type Conversion1 : DataTypeConversion  OutDataTypeStr=uint8  SaturateOnIntegerOverflow=off  RndMeth=Floor
  Data Type Conversion2 : DataTypeConversion  OutDataTypeStr=uint8  SaturateOnIntegerOverflow=off  RndMeth=Floor
  Data Type Conversion3 : DataTypeConversion  OutDataTypeStr=uint8  SaturateOnIntegerOverflow=off  RndMeth=Floor
  Divide : Product  Inputs=*/  OutDataTypeStr=int16
  Divide1 : Product  Inputs=*/  OutDataTypeStr=int16
  Ground10 : Constant  Value=48  OutDataTypeStr=int16
  Ground8 : Constant  Value=100  OutDataTypeStr=int16
  Ground9 : Constant  Value=10  OutDataTypeStr=int16
  Math Function1 : Math  Operator=rem  SignedPower=on
  Math Function2 : Math  Operator=rem  SignedPower=on
  Mux3 : Mux  Inputs=3
  Saturation1 : Saturate  UpperLimit=999  LowerLimit=0  OutDataTypeStr=int16
  Saturation2 : Saturate  UpperLimit=9  LowerLimit=0
  Sum1 : Sum  OutDataTypeStr=uint8
  Sum2 : Sum  Inputs=+-  OutDataTypeStr=double
  Sum3 : Sum  Inputs=+-
  Sum4 : Sum  OutDataTypeStr=uint8
  Sum6 : Sum  OutDataTypeStr=uint8
  Out1 : Outport
  wires:
  Saturation1/1 -> Sum2/1, Math Function1/1
  Ground8/1 -> Divide/2, Math Function1/2
  Sum4/1 -> Data Type Conversion2/1
  Sum1/1 -> Data Type Conversion3/1
  Divide/1 -> Sum4/1
  Divide1/1 -> Sum6/1
  Sum2/1 -> Divide/1
  In1/1 -> Saturation1/1
  Data Type Conversion2/1 -> Mux3/1
  Mux3/1 -> Out1/1
  Data Type Conversion3/1 -> Mux3/3
  Data Type Conversion1/1 -> Mux3/2
  Math Function1/1 -> Sum2/2, Math Function2/1, Sum3/1
  Sum3/1 -> Divide1/1
  Sum6/1 -> Data Type Conversion1/1
  Ground10/1 -> Sum4/2, Sum6/2, Sum1/1
  Ground9/1 -> Divide1/2, Math Function2/2
  Math Function2/1 -> Sum3/2, Saturation2/1
  Saturation2/1 -> Sum1/2

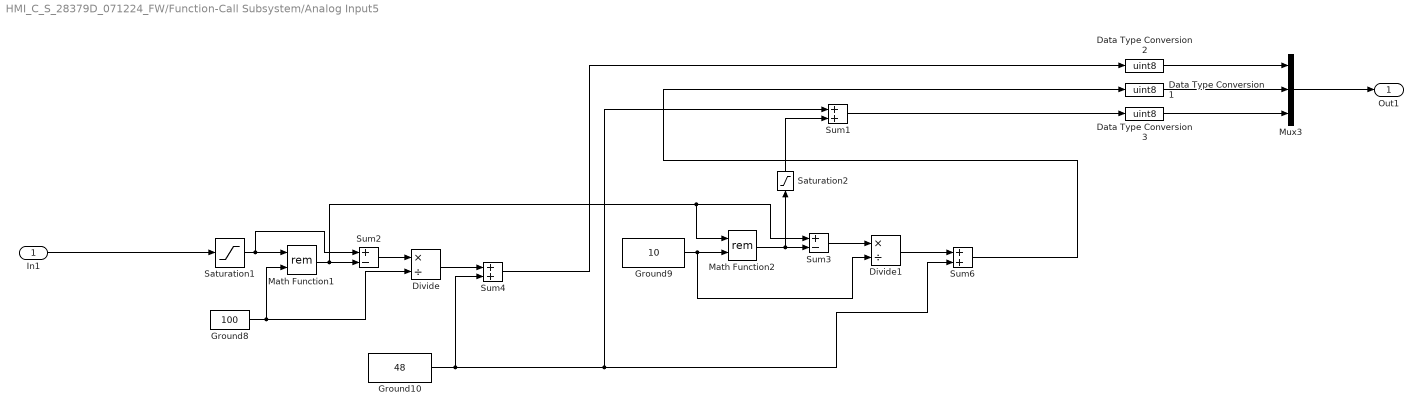
== system HMI_C_S_28379D_071224_FW/Function-Call Subsystem/Analog Input5 ==
  In1 : Inport
  Data Type Conversion1 : DataTypeConversion  OutDataTypeStr=uint8  SaturateOnIntegerOverflow=off  RndMeth=Floor
  Data Type Conversion2 : DataTypeConversion  OutDataTypeStr=uint8  SaturateOnIntegerOverflow=off  RndMeth=Floor
  Data Type Conversion3 : DataTypeConversion  OutDataTypeStr=uint8  SaturateOnIntegerOverflow=off  RndMeth=Floor
  Divide : Product  Inputs=*/  OutDataTypeStr=int16
  Divide1 : Product  Inputs=*/  OutDataTypeStr=int16
  Ground10 : Constant  Value=48  OutDataTypeStr=int16
  Ground8 : Constant  Value=100  OutDataTypeStr=int16
  Ground9 : Constant  Value=10  OutDataTypeStr=int16
  Math Function1 : Math  Operator=rem  SignedPower=on
  Math Function2 : Math  Operator=rem  SignedPower=on
  Mux3 : Mux  Inputs=3
  Saturation1 : Saturate  UpperLimit=999  LowerLimit=0  OutDataTypeStr=int16
  Saturation2 : Saturate  UpperLimit=9  LowerLimit=0
  Sum1 : Sum  OutDataTypeStr=uint8
  Sum2 : Sum  Inputs=+-  OutDataTypeStr=double
  Sum3 : Sum  Inputs=+-
  Sum4 : Sum  OutDataTypeStr=uint8
  Sum6 : Sum  OutDataTypeStr=uint8
  Out1 : Outport
  wires:
  Saturation1/1 -> Sum2/1, Math Function1/1
  Ground8/1 -> Divide/2, Math Function1/2
  Sum4/1 -> Data Type Conversion2/1
  Sum1/1 -> Data Type Conversion3/1
  Divide/1 -> Sum4/1
  Divide1/1 -> Sum6/1
  Sum2/1 -> Divide/1
  In1/1 -> Saturation1/1
  Data Type Conversion2/1 -> Mux3/1
  Mux3/1 -> Out1/1
  Data Type Conversion3/1 -> Mux3/3
  Data Type Conversion1/1 -> Mux3/2
  Math Function1/1 -> Sum2/2, Math Function2/1, Sum3/1
  Sum3/1 -> Divide1/1
  Sum6/1 -> Data Type Conversion1/1
  Ground10/1 -> Sum4/2, Sum6/2, Sum1/1
  Ground9/1 -> Divide1/2, Math Function2/2
  Math Function2/1 -> Sum3/2, Saturation2/1
  Saturation2/1 -> Sum1/2

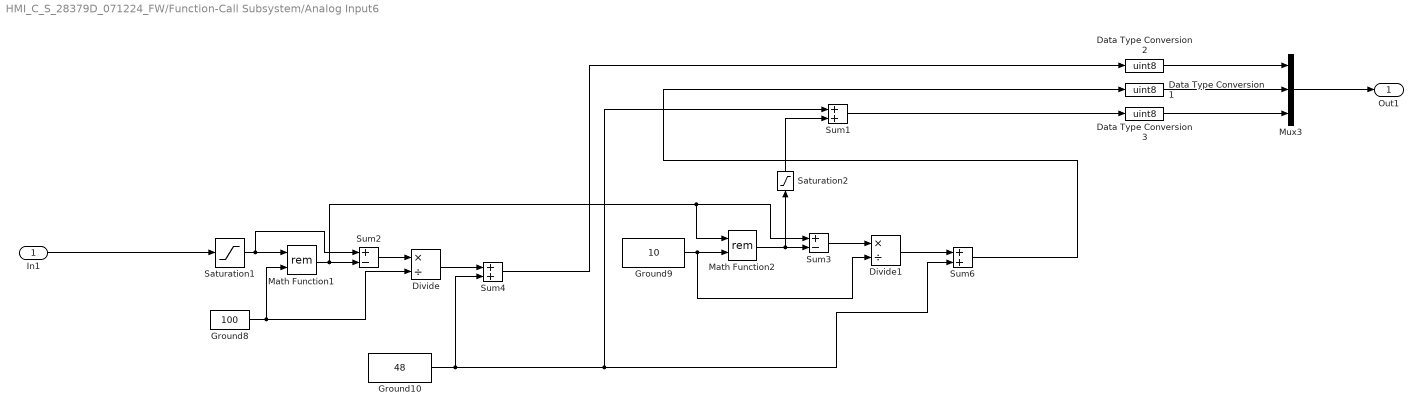
== system HMI_C_S_28379D_071224_FW/Function-Call Subsystem/Analog Input6 ==
  In1 : Inport
  Data Type Conversion1 : DataTypeConversion  OutDataTypeStr=uint8  SaturateOnIntegerOverflow=off  RndMeth=Floor
  Data Type Conversion2 : DataTypeConversion  OutDataTypeStr=uint8  SaturateOnIntegerOverflow=off  RndMeth=Floor
  Data Type Conversion3 : DataTypeConversion  OutDataTypeStr=uint8  SaturateOnIntegerOverflow=off  RndMeth=Floor
  Divide : Product  Inputs=*/  OutDataTypeStr=int16
  Divide1 : Product  Inputs=*/  OutDataTypeStr=int16
  Ground10 : Constant  Value=48  OutDataTypeStr=int16
  Ground8 : Constant  Value=100  OutDataTypeStr=int16
  Ground9 : Constant  Value=10  OutDataTypeStr=int16
  Math Function1 : Math  Operator=rem  SignedPower=on
  Math Function2 : Math  Operator=rem  SignedPower=on
  Mux3 : Mux  Inputs=3
  Saturation1 : Saturate  UpperLimit=999  LowerLimit=0  OutDataTypeStr=int16
  Saturation2 : Saturate  UpperLimit=9  LowerLimit=0
  Sum1 : Sum  OutDataTypeStr=uint8
  Sum2 : Sum  Inputs=+-  OutDataTypeStr=double
  Sum3 : Sum  Inputs=+-
  Sum4 : Sum  OutDataTypeStr=uint8
  Sum6 : Sum  OutDataTypeStr=uint8
  Out1 : Outport
  wires:
  Saturation1/1 -> Sum2/1, Math Function1/1
  Ground8/1 -> Divide/2, Math Function1/2
  Sum4/1 -> Data Type Conversion2/1
  Sum1/1 -> Data Type Conversion3/1
  Divide/1 -> Sum4/1
  Divide1/1 -> Sum6/1
  Sum2/1 -> Divide/1
  In1/1 -> Saturation1/1
  Data Type Conversion2/1 -> Mux3/1
  Mux3/1 -> Out1/1
  Data Type Conversion3/1 -> Mux3/3
  Data Type Conversion1/1 -> Mux3/2
  Math Function1/1 -> Sum2/2, Math Function2/1, Sum3/1
  Sum3/1 -> Divide1/1
  Sum6/1 -> Data Type Conversion1/1
  Ground10/1 -> Sum4/2, Sum6/2, Sum1/1
  Ground9/1 -> Divide1/2, Math Function2/2
  Math Function2/1 -> Sum3/2, Saturation2/1
  Saturation2/1 -> Sum1/2

== system HMI_C_S_28379D_071224_FW/Function-Call Subsystem/Analog Input7 ==
  In1 : Inport
  Data Type Conversion1 : DataTypeConversion  OutDataTypeStr=uint8  SaturateOnIntegerOverflow=off  RndMeth=Floor
  Data Type Conversion2 : DataTypeConversion  OutDataTypeStr=uint8  SaturateOnIntegerOverflow=off  RndMeth=Floor
  Data Type Conversion3 : DataTypeConversion  OutDataTypeStr=uint8  SaturateOnIntegerOverflow=off  RndMeth=Floor
  Divide : Product  Inputs=*/  OutDataTypeStr=int16
  Divide1 : Product  Inputs=*/  OutDataTypeStr=int16
  Ground10 : Constant  Value=48  OutDataTypeStr=int16
  Ground8 : Constant  Value=100  OutDataTypeStr=int16
  Ground9 : Constant  Value=10  OutDataTypeStr=int16
  Math Function1 : Math  Operator=rem  SignedPower=on
  Math Function2 : Math  Operator=rem  SignedPower=on
  Mux3 : Mux  Inputs=3
  Saturation1 : Saturate  UpperLimit=999  LowerLimit=0  OutDataTypeStr=int16
  Saturation2 : Saturate  UpperLimit=9  LowerLimit=0
  Sum1 : Sum  OutDataTypeStr=uint8
  Sum2 : Sum  Inputs=+-  OutDataTypeStr=double
  Sum3 : Sum  Inputs=+-
  Sum4 : Sum  OutDataTypeStr=uint8
  Sum6 : Sum  OutDataTypeStr=uint8
  Out1 : Outport
  wires:
  Saturation1/1 -> Sum2/1, Math Function1/1
  Ground8/1 -> Divide/2, Math Function1/2
  Sum4/1 -> Data Type Conversion2/1
  Sum1/1 -> Data Type Conversion3/1
  Divide/1 -> Sum4/1
  Divide1/1 -> Sum6/1
  Sum2/1 -> Divide/1
  In1/1 -> Saturation1/1
  Data Type Conversion2/1 -> Mux3/1
  Mux3/1 -> Out1/1
  Data Type Conversion3/1 -> Mux3/3
  Data Type Conversion1/1 -> Mux3/2
  Math Function1/1 -> Sum2/2, Math Function2/1, Sum3/1
  Sum3/1 -> Divide1/1
  Sum6/1 -> Data Type Conversion1/1
  Ground10/1 -> Sum4/2, Sum6/2, Sum1/1
  Ground9/1 -> Divide1/2, Math Function2/2
  Math Function2/1 -> Sum3/2, Saturation2/1
  Saturation2/1 -> Sum1/2

== system HMI_C_S_28379D_071224_FW/Function-Call Subsystem/Analog Input8 ==
  In1 : Inport
  Data Type Conversion1 : DataTypeConversion  OutDataTypeStr=uint8  SaturateOnIntegerOverflow=off  RndMeth=Floor
  Data Type Conversion2 : DataTypeConversion  OutDataTypeStr=uint8  SaturateOnIntegerOverflow=off  RndMeth=Floor
  Data Type Conversion3 : DataTypeConversion  OutDataTypeStr=uint8  SaturateOnIntegerOverflow=off  RndMeth=Floor
  Divide : Product  Inputs=*/  OutDataTypeStr=int16
  Divide1 : Product  Inputs=*/  OutDataTypeStr=int16
  Ground10 : Constant  Value=48  OutDataTypeStr=int16
  Ground8 : Constant  Value=100  OutDataTypeStr=int16
  Ground9 : Constant  Value=10  OutDataTypeStr=int16
  Math Function1 : Math  Operator=rem  SignedPower=on
  Math Function2 : Math  Operator=rem  SignedPower=on
  Mux3 : Mux  Inputs=3
  Saturation1 : Saturate  UpperLimit=999  LowerLimit=0  OutDataTypeStr=int16
  Saturation2 : Saturate  UpperLimit=9  LowerLimit=0
  Sum1 : Sum  OutDataTypeStr=uint8
  Sum2 : Sum  Inputs=+-  OutDataTypeStr=double
  Sum3 : Sum  Inputs=+-
  Sum4 : Sum  OutDataTypeStr=uint8
  Sum6 : Sum  OutDataTypeStr=uint8
  Out1 : Outport
  wires:
  Saturation1/1 -> Sum2/1, Math Function1/1
  Ground8/1 -> Divide/2, Math Function1/2
  Sum4/1 -> Data Type Conversion2/1
  Sum1/1 -> Data Type Conversion3/1
  Divide/1 -> Sum4/1
  Divide1/1 -> Sum6/1
  Sum2/1 -> Divide/1
  In1/1 -> Saturation1/1
  Data Type Conversion2/1 -> Mux3/1
  Mux3/1 -> Out1/1
  Data Type Conversion3/1 -> Mux3/3
  Data Type Conversion1/1 -> Mux3/2
  Math Function1/1 -> Sum2/2, Math Function2/1, Sum3/1
  Sum3/1 -> Divide1/1
  Sum6/1 -> Data Type Conversion1/1
  Ground10/1 -> Sum4/2, Sum6/2, Sum1/1
  Ground9/1 -> Divide1/2, Math Function2/2
  Math Function2/1 -> Sum3/2, Saturation2/1
  Saturation2/1 -> Sum1/2

== system HMI_C_S_28379D_071224_FW/Function-Call Subsystem/Analog Input9 ==
  In1 : Inport
  Data Type Conversion1 : DataTypeConversion  OutDataTypeStr=uint8  SaturateOnIntegerOverflow=off  RndMeth=Floor
  Data Type Conversion2 : DataTypeConversion  OutDataTypeStr=uint8  SaturateOnIntegerOverflow=off  RndMeth=Floor
  Data Type Conversion3 : DataTypeConversion  OutDataTypeStr=uint8  SaturateOnIntegerOverflow=off  RndMeth=Floor
  Divide : Product  Inputs=*/  OutDataTypeStr=int16
  Divide1 : Product  Inputs=*/  OutDataTypeStr=int16
  Ground10 : Constant  Value=48  OutDataTypeStr=int16
  Ground8 : Constant  Value=100  OutDataTypeStr=int16
  Ground9 : Constant  Value=10  OutDataTypeStr=int16
  Math Function1 : Math  Operator=rem  SignedPower=on
  Math Function2 : Math  Operator=rem  SignedPower=on
  Mux3 : Mux  Inputs=3
  Saturation1 : Saturate  UpperLimit=999  LowerLimit=0  OutDataTypeStr=int16
  Saturation2 : Saturate  UpperLimit=9  LowerLimit=0
  Sum1 : Sum  OutDataTypeStr=uint8
  Sum2 : Sum  Inputs=+-  OutDataTypeStr=double
  Sum3 : Sum  Inputs=+-
  Sum4 : Sum  OutDataTypeStr=uint8
  Sum6 : Sum  OutDataTypeStr=uint8
  Out1 : Outport
  wires:
  Saturation1/1 -> Sum2/1, Math Function1/1
  Ground8/1 -> Divide/2, Math Function1/2
  Sum4/1 -> Data Type Conversion2/1
  Sum1/1 -> Data Type Conversion3/1
  Divide/1 -> Sum4/1
  Divide1/1 -> Sum6/1
  Sum2/1 -> Divide/1
  In1/1 -> Saturation1/1
  Data Type Conversion2/1 -> Mux3/1
  Mux3/1 -> Out1/1
  Data Type Conversion3/1 -> Mux3/3
  Data Type Conversion1/1 -> Mux3/2
  Math Function1/1 -> Sum2/2, Math Function2/1, Sum3/1
  Sum3/1 -> Divide1/1
  Sum6/1 -> Data Type Conversion1/1
  Ground10/1 -> Sum4/2, Sum6/2, Sum1/1
  Ground9/1 -> Divide1/2, Math Function2/2
  Math Function2/1 -> Sum3/2, Saturation2/1
  Saturation2/1 -> Sum1/2

== system HMI_C_S_28379D_071224_FW/Function-Call Subsystem/Digital Input2 ==
  Start_sw_Status : Inport
  Ground10 : Constant  Value=48  OutDataTypeStr=int16
  Saturation1 : Saturate  UpperLimit=1  LowerLimit=0  OutDataTypeStr=double
  Sum4 : Sum  OutDataTypeStr=uint8
  Input : Outport
  wires:
  Saturation1/1 -> Sum4/1
  Start_sw_Status/1 -> Saturation1/1
  Ground10/1 -> Sum4/2
  Sum4/1 -> Input/1

== system HMI_C_S_28379D_071224_FW/Subsystem/Subsystem ==
  In1 : Inport
  In2 : Inport  Port=2
  In3 : Inport  Port=3
  Data Type Conversion : DataTypeConversion  OutDataTypeStr=single  SaturateOnIntegerOverflow=off  RndMeth=Floor
  Multiply1 : Gain
  Multiply2 : Gain  Gain=1/10
  Multiply4 : Gain  Gain=1/10
  P17 : DataTypeConversion  OutDataTypeStr=uint8  SaturateOnIntegerOverflow=off  RndMeth=Floor
  P19 : DataTypeConversion  OutDataTypeStr=uint8  SaturateOnIntegerOverflow=off  RndMeth=Floor
  P21 : DataTypeConversion  OutDataTypeStr=uint8  SaturateOnIntegerOverflow=off  RndMeth=Floor
  Sum18 : Sum  Inputs=|++
  Terminator3 : Terminator
  Out1 : Outport
  wires:
  Multiply2/1 -> Terminator3/1
  In3/1 -> P17/1
  P21/1 -> Multiply1/1
  P19/1 -> Multiply2/1
  Data Type Conversion/1 -> Sum18/2
  In1/1 -> P21/1
  Multiply4/1 -> Data Type Conversion/1
  Multiply1/1 -> Sum18/1
  P17/1 -> Multiply4/1
  In2/1 -> P19/1
  Sum18/1 -> Out1/1

== system HMI_C_S_28379D_071224_FW/Subsystem/Subsystem1 ==
  In1 : Inport
  In2 : Inport  Port=2
  In3 : Inport  Port=3
  Data Type Conversion : DataTypeConversion  OutDataTypeStr=single  SaturateOnIntegerOverflow=off  RndMeth=Floor
  Multiply1 : Gain
  Multiply2 : Gain  Gain=1/10
  Multiply4 : Gain  Gain=1/10
  P17 : DataTypeConversion  OutDataTypeStr=uint8  SaturateOnIntegerOverflow=off  RndMeth=Floor
  P19 : DataTypeConversion  OutDataTypeStr=uint8  SaturateOnIntegerOverflow=off  RndMeth=Floor
  P21 : DataTypeConversion  OutDataTypeStr=uint8  SaturateOnIntegerOverflow=off  RndMeth=Floor
  Sum18 : Sum  Inputs=|++
  Terminator3 : Terminator
  Out1 : Outport
  wires:
  Multiply2/1 -> Terminator3/1
  In3/1 -> P17/1
  P21/1 -> Multiply1/1
  P19/1 -> Multiply2/1
  Data Type Conversion/1 -> Sum18/2
  In1/1 -> P21/1
  Multiply4/1 -> Data Type Conversion/1
  Multiply1/1 -> Sum18/1
  P17/1 -> Multiply4/1
  In2/1 -> P19/1
  Sum18/1 -> Out1/1

== matlab function HMI_C_S_28379D_071224_FW/Subsystem/MATLAB Function1 ==
  data: input2 input; Output1 output
function Output1 = fcn(input2)
% function y = fcn(u)
% 
% y = u;
% function Output1  = unBuf(input1)
% % %#codegen
% % % Declare input as a string and output as an integer
coder.cinclude('stdlib.h'); % Include the standard C library
Output1 = single(0);  % Initialize output as 32-bit integer
 Output1 = coder.ceval('atof', input2(:,1)); % Call the C atoi function
% % 
% Output2 = double(0); % Initialize output as 32-bit integer
% Output2 = coder.ceval('atof', input2(:,1)); % Call the C atoi function
% 
% Output3 = double(0); % Initialize output as 32-bit integer
% Output3 = coder.ceval('atof', input(:,3)); % Call the C atoi function
% 
% Output4 = double(0); % Initialize output as 32-bit integer
% Output4 = coder.ceval('atof', input(:,4)); % Call the C atoi function
% 
% Output5 = double(0); % Initialize output as 32-bit integer
% Output5 = coder.ceval('atof', input(:,5)); % Call the C atoi function



%#codegen
% Declare input as a string and output as a double
%  coder.cinclude('stdlib.h'); % Include the standard C library
% 
% Output1 = coder.ceval('atof', input2(:,1))); % Call the C atof function and cast to double

% Output1 = single(coder.ceval('atof', input2(:,1)))
% Output1 = coder.ceval('atof', input2(:,1)); % Call the C atof function and cast to double
% % Output3 =coder.ceval('atof', input(:,3))); % Call the C atof function and cast to double
% Output4 = coder.ceval('atof', input(:,4))); % Call the C atof function and cast to double
% Output5 = coder.ceval('atof', input(:,5))); % Call the C atof function and cast to double


end
